simulink model "BD11"  (R2017a)
settings: Solver=ode45  StartTime=0.0  StopTime=50  RelTol=1e-3  EnableMultiTasking=on
settings Model: Creator=Usman Arshad  LastModifiedBy=John
settings DataIOCC: LimitDataPoints=on  SaveFormat=Array
settings OptimizationCC: LifeSpan=inf
settings DebuggingCC: SolverPrmCheckMsg=warning  SFUnexpectedBacktrackingDiag=warning  SFNoUnconditionalDefaultTransitionDiag=warning  SFExecutionAtInitializationDiag=none
settings HardwareCC: ProdBitPerPointer=32  ProdBitPerSizeT=32  ProdBitPerPtrDiffT=32  ProdLargestAtomicFloat=None  ProdIntDivRoundTo=Undefined  ProdEndianess=Unspecified  ProdWordSize=32  ProdHWDeviceType=32-bit Generic
settings ModelReferenceCC: PropagateSignalLabelsOutOfModel=off
settings GRTTargetCC: TargetLangStandard=C89/C90 (ANSI)  GeneratePreprocessorConditionals=Disable all
settings ConfigComp: CovMetricSettings=dw  CovHtmlReporting=on  CovSaveCumulativeToWorkspaceVar=on  CovSaveSingleToWorkspaceVar=on  CovExternalEMLEnable=off  CovSFcnEnable=off

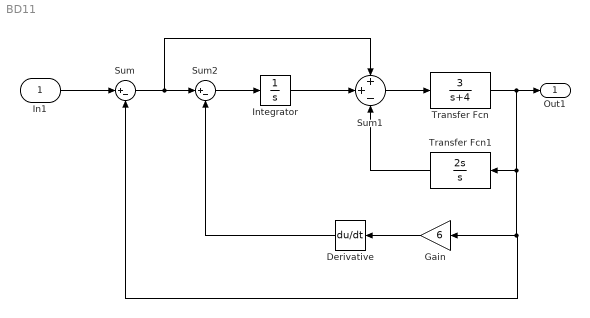
== system BD11 ==
  In1 : Inport
  Derivative : Derivative
  Gain : Gain  Gain=6
  Integrator : Integrator
  Sum : Sum  Inputs=|+-
  Sum1 : Sum  Inputs=++-
  Sum2 : Sum  Inputs=|+-
  Transfer Fcn : TransferFcn  Numerator=[3]  Denominator=[1 4]
  Transfer Fcn1 : TransferFcn  Numerator=[2,0]  Denominator=[1 0]
  Out1 : Outport
  wires:
  In1/1 -> Sum/1
  Sum2/1 -> Integrator/1
  Integrator/1 -> Sum1/2
  Sum/1 -> Sum1/1, Sum2/1
  Sum1/1 -> Transfer Fcn/1
  Transfer Fcn1/1 -> Sum1/3
  Gain/1 -> Derivative/1
  Derivative/1 -> Sum2/2
  Transfer Fcn/1 -> Out1/1, Gain/1, Sum/2, Transfer Fcn1/1
